simulink model "gm_nco"  (R2023a)
settings: Solver=VariableStepAuto  StartTime=0.0  StopTime=20480  RelTol=1e-3
undefined symbols (not defined in the file or in its folder): hbi
libraries: dsphdlfiltering2 x1, dsphdlsigops2 x1
settings Model: Creator=31651  LastModifiedBy=31651
settings OptimizationCC: BlockReduction=off  ConditionallyExecuteInputs=off  DefaultParameterBehavior=Inlined
settings DebuggingCC: AlgebraicLoopMsg=error  InheritedTsInSrcMsg=none
settings HardwareCC: ProdBitPerPointer=32  ProdBitPerSizeT=32  ProdBitPerPtrDiffT=32  ProdLargestAtomicFloat=None  ProdIntDivRoundTo=Undefined  ProdEndianess=Unspecified  ProdWordSize=32  ProdHWDeviceType=ASIC/FPGA->ASIC/FPGA  TargetBitPerPointer=64  TargetBitPerSizeT=64  TargetBitPerPtrDiffT=64  TargetLongLongMode=on  TargetIntDivRoundTo=Zero  TargetEndianess=LittleEndian  TargetWordSize=64  TargetHWDeviceType=Custom Processor->MATLAB Host Computer  ProdEqTarget=off

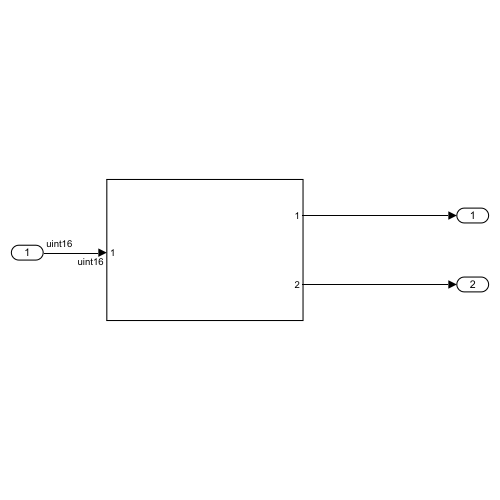
[thumbnail: Simulink's stored preview of the top-level diagram]
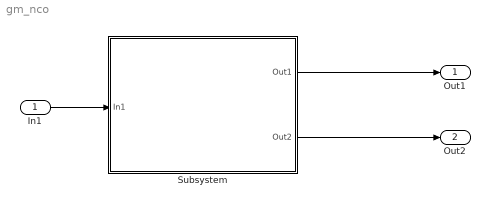
== system gm_nco ==
  In1 : Inport  OutDataTypeStr=uint16  PortDimensions=1  SampleTime=1
  Subsystem : Subsystem
  Out1 : Outport  SampleTime=1  VectorParamsAs1DForOutWhenUnconnected=off
  Out2 : Outport  Port=2  SampleTime=1  VectorParamsAs1DForOutWhenUnconnected=off
  wires:
  In1/1 -> Subsystem/1(In1)
  Subsystem/1(Out1) -> Out1/1
  Subsystem/2(Out2) -> Out2/1

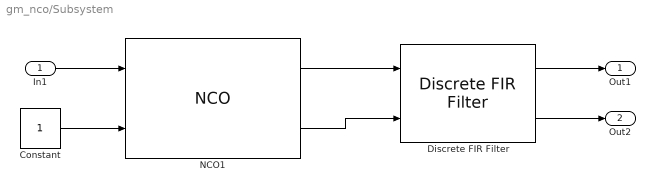
== system gm_nco/Subsystem ==
  In1 : Inport  OutDataTypeStr=uint16  PortDimensions=1  SampleTime=1
  Constant : Constant  VectorParams1D=off  OutDataTypeStr=boolean  SampleTime=1
  Discrete FIR Filter : dsphdlfiltering2/Discrete FIR Filter  NumeratorSource=Property  Numerator=hbi  NumeratorPrototype=[]  FilterStructure=Direct form systolic  SerializationOption=Minimum number of cycles between valid input samples  NumCycles=2  NumberOfMultipliers=2  SimulateUsing=Code generation  roundingMode=Floor  overflowMode=off  CoefficientsDataTypeStr=Inherit: Same word length as input  OutputDataTypeStr=Inherit: Same word length as input  ResetInputPort=off  HDLGlobalReset=off
  NCO1 : dsphdlsigops2/NCO  PhaseIncrementSource=Input port  PhaseIncrement=3200  PhaseOffsetSource=Property  PhaseOffset=0  DitherSource=Property  NumDitherBits=4  SamplesPerFrame=1  LUTCompress=off  ResetAction=off  Waveform=Sine  PhasePort=off  SimulateUsing=Code generation  AccumulatorWL=16  PhaseQuantization=on  NumQuantizerAccumulatorBits=12  OutputDataType=Binary point scaling  OutputWL=16  OutputFL=14
  Out1 : Outport  SampleTime=1
  Out2 : Outport  Port=2  SampleTime=1
  wires:
  In1/1 -> NCO1/1
  Constant/1 -> NCO1/2
  Discrete FIR Filter/1 -> Out1/1
  Discrete FIR Filter/2 -> Out2/1
  NCO1/1 -> Discrete FIR Filter/1
  NCO1/2 -> Discrete FIR Filter/2
